simulink model "RT_AI_3"  (R2024b)
settings: Solver=ode1  StartTime=0.0  StopTime=3  FixedStep=Ts  RelTol=1e-3
PreLoadFcn:
  | Net_improve_init;L=Lac_MV;Tctrl=Ts;
PostLoadFcn:
  | Net_improve_init;L=Lac_MV;Tctrl=Ts;
InitFcn:
  | Net_improve_init;L=Lac_MV;Tctrl=Ts;
values from neighbouring files (symbols this model uses):
  C1 = 3300e-6    (= 0.0033)    [Net_improve_init.m]
  f_cari = 2e4/4.1    (= 4878.04878049)    [Net_improve_init.m]
  fs = 50    [Net_improve_init.m]
  Lac_MV = 0.005*3    (= 0.015)    [Net_improve_init.m]
  Pref = 14e3    (= 14000)    [Net_improve_init.m]
  Rac_MV = 0.1    [Net_improve_init.m]
  Ts = 20e-6    (= 2e-05)    [Net_improve_init.m]
  Vac_peak_MV = 220*sqrt(2)    [Net_improve_init.m]
  Vdc = 720    [Net_improve_init.m]
undefined symbols (not defined in the file or in its folder): dend, DiscIntNeverNeededParam, eHSx64gen4_PMSMSH_with_IOs, EX, numd, TE0741_4
libraries: rtlab x6, spsControlledVoltageSourceLib x6, powerlib_extras x5, artemis x3, spsControlledCurrentSourceLib x3, rtio_opalrt_common x3, spsGroundLib x3, simulink x3, spsCurrentMeasurementLib x2, spsThreePhaseVIMeasurementLib x1, spsIdealSwitchLib x1, spsPower3phInstantaneousLib x1
(part 2 of 2)

== matlab function RT_AI_3/SM_AI/MATLAB Function1 ==
  settings: updateMethod=DISCRETE
  data: u input; dz output
function dz = phnode_forward(u)
    % =========================================================
    % 0. Persistent variables: load weights only once
    % =========================================================
    persistent W00 b00 W01 b01 W10 b10 W11 b11 W2 b2 p

    if isempty(W00)

        w = coder.load('3level_pHNODE_weights.mat');

        % =====================================================
        % R_3level MLP: input 17 -> hidden 16 -> hidden 16 -> output 5
        % Each hidden block: Linear -> LayerNorm -> SiLU
        % =====================================================
        W00 = double(w.R_module_net_0_0_weight);
        b00 = double(w.R_module_net_0_0_bias(:));
        W01 = double(w.R_module_net_0_1_weight(:));
        b01 = double(w.R_module_net_0_1_bias(:));

        W10 = double(w.R_module_net_1_0_weight);
        b10 = double(w.R_module_net_1_0_bias(:));
        W11 = double(w.R_module_net_1_1_weight(:));
        b11 = double(w.R_module_net_1_1_bias(:));

        W2  = double(w.R_module_net_2_weight);
        b2  = double(w.R_module_net_2_bias(:));

        % =====================================================
        % P^{-1}_3level
        % P^{-1} = diag(1/Cp, 1/Cn, 1/La, 1/Lb, 1/Lc)
        % =====================================================
        p_raw = double(w.Pinv_module_p_raw(:));

        base_scale = [
            1/3.3e-3;
            1/3.3e-3;
            1/0.015;
            1/0.015;
            1/0.015
        ];

        p = log(1.0 + exp(p_raw)) .* base_scale;
    end

    % =========================================================
    % 1. Split input vector
    %
    % u = [
    %   z(1:5);
    %   u_ext(1:5);
    %   u_sw(1:12)
    % ]
    %
    % z     = [vcp, vcn, ia, ib, ic]
    % u_ext = [idcp, idcn, ea, eb, ec]
    % u_sw  = [
    %   Sa1, Sa2, Sa3, Sa4,
    %   Sb1, Sb2, Sb3, Sb4,
    %   Sc1, Sc2, Sc3, Sc4
    % ]
    % =========================================================
    z     = double(u(1:5));
    u_ext = double(u(6:10));
    u_sw  = double(u(11:22));

    % =========================================================
    % 2. Compute dissipation vector R_theta
    % =========================================================
    h = [z; u_sw];

    % ---------------- Block 0 ----------------
    h = W00 * h + b00;

    mu = mean(h);
    var_h = mean((h - mu).^2);
    h = (h - mu) ./ sqrt(var_h + 1e-5);

    h = W01 .* h + b01;
    h = h ./ (1 + exp(-h));     % SiLU

    % ---------------- Block 1 ----------------
    h = W10 * h + b10;

    mu = mean(h);
    var_h = mean((h - mu).^2);
    h = (h - mu) ./ sqrt(var_h + 1e-5);

    h = W11 .* h + b11;
    h = h ./ (1 + exp(-h));     % SiLU

    % ---------------- Output Linear ----------------
    r_out = W2 * h + b2;
    r_full = log(1.0 + exp(r_out));    % Softplus

    % =========================================================
    % 3. Build three-level switching-induced Jz
    %
    % M(s) = [
    %   Sa1*Sa2     Sb1*Sb2     Sc1*Sc2
    %  -Sa3*Sa4    -Sb3*Sb4    -Sc3*Sc4
    % ]
    %
    % J = [ 0   M
    %      -M'  0 ]
    % =========================================================
    Sa1 = u_sw(1);
    Sa2 = u_sw(2);
    Sa3 = u_sw(3);
    Sa4 = u_sw(4);

    Sb1 = u_sw(5);
    Sb2 = u_sw(6);
    Sb3 = u_sw(7);
    Sb4 = u_sw(8);

    Sc1 = u_sw(9);
    Sc2 = u_sw(10);
    Sc3 = u_sw(11);
    Sc4 = u_sw(12);

    ma_p = Sa1 * Sa2;
    mb_p = Sb1 * Sb2;
    mc_p = Sc1 * Sc2;

    ma_n = Sa3 * Sa4;
    mb_n = Sb3 * Sb4;
    mc_n = Sc3 * Sc4;

    Jz = zeros(5, 1, 'double');

    Jz(1) =  ma_p * z(3) + mb_p * z(4) + mc_p * z(5);
    Jz(2) = -ma_n * z(3) - mb_n * z(4) - mc_n * z(5);

    Jz(3) = -ma_p * z(1) + ma_n * z(2);
    Jz(4) = -mb_p * z(1) + mb_n * z(2);
    Jz(5) = -mc_p * z(1) + mc_n * z(2);

    % =========================================================
    % 4. dz/dt = P^{-1} [ Jz - Rz + u_ext ]
    % =========================================================
    rhs = Jz - r_full .* z + u_ext;

    dz = p .* rhs;
end
